simulink model "untitled"  (R2018b)
settings: Solver=ode5  StartTime=0.0  StopTime=10.0  FixedStep=0.2  RelTol=1e-3
settings Model: Creator=root  LastModifiedBy=root

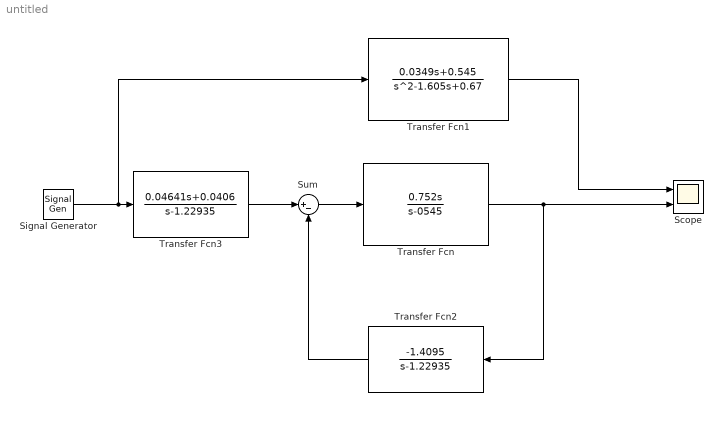
== system untitled ==
  Scope : Scope  NumInputPorts=2
  Signal Generator : SignalGenerator  WaveForm=square  Units=rad/sec
  Sum : Sum  Inputs=|+-
  Transfer Fcn : TransferFcn  Numerator=[0.752 0]  Denominator=[1 -0545]
  Transfer Fcn1 : TransferFcn  Numerator=[0.0349 0.545]  Denominator=[1 -1.605 0.67]
  Transfer Fcn2 : TransferFcn  Numerator=[-1.4095 ]  Denominator=[1 -1.22935]
  Transfer Fcn3 : TransferFcn  Numerator=[0.04641 0.0406]  Denominator=[1 -1.22935]
  wires:
  Transfer Fcn3/1 -> Sum/1
  Sum/1 -> Transfer Fcn/1
  Transfer Fcn/1 -> Transfer Fcn2/1, Scope/2
  Transfer Fcn2/1 -> Sum/2
  Signal Generator/1 -> Transfer Fcn1/1, Transfer Fcn3/1
  Transfer Fcn1/1 -> Scope/1
